simulink model "CrashTest"  (R2024a)
settings: Solver=VariableStepAuto  StartTime=0.0  StopTime=Inf  RelTol=1e-3
model workspace (MAT data in the model file):
  SL_ROS_VariableLengthArrays_MaxSizes.CommonInfo.ArrayTruncateAction = 'EmitWarning'
  SL_ROS_VariableLengthArrays_MaxSizes.MsgTypeMap = containers.Map
  SL_ROS_VariableLengthArrays_MaxSizes.MsgTypeMap.serialization.keys = {'sensor_msgs/PointCloud2', 'sensor_msgs/PointField'}
  SL_ROS_VariableLengthArrays_MaxSizes.MsgTypeMap.serialization.values{1}(1).PropertyName = 'Data'
  SL_ROS_VariableLengthArrays_MaxSizes.MsgTypeMap.serialization.values{1}(1).DataType = 'uint8'
  SL_ROS_VariableLengthArrays_MaxSizes.MsgTypeMap.serialization.values{1}(1).MaxLength = 1000000
  SL_ROS_VariableLengthArrays_MaxSizes.MsgTypeMap.serialization.values{1}(2).PropertyName = 'Fields'
  SL_ROS_VariableLengthArrays_MaxSizes.MsgTypeMap.serialization.values{1}(2).DataType = 'sensor_msgs/PointField'
  SL_ROS_VariableLengthArrays_MaxSizes.MsgTypeMap.serialization.values{1}(2).MaxLength = 16
  SL_ROS_VariableLengthArrays_MaxSizes.MsgTypeMap.serialization.values{2}.PropertyName = 'Name'
  SL_ROS_VariableLengthArrays_MaxSizes.MsgTypeMap.serialization.values{2}.DataType = 'uint8'
  SL_ROS_VariableLengthArrays_MaxSizes.MsgTypeMap.serialization.values{2}.MaxLength = 1000000
  SL_ROS_VariableLengthArrays_MaxSizes.MsgTypeMap.serialization.uniformity = 0
  SL_ROS_VariableLengthArrays_MaxSizes.MsgTypeMap.serialization.keyType = 'char'
  SL_ROS_VariableLengthArrays_MaxSizes.MsgTypeMap.serialization.valueType = 'any'
libraries: robotlib x4, visionsinks x1
settings Model: Creator=lajos  LastModifiedBy=Fahim
settings RTWCC: GPUComputeCapability=3.5

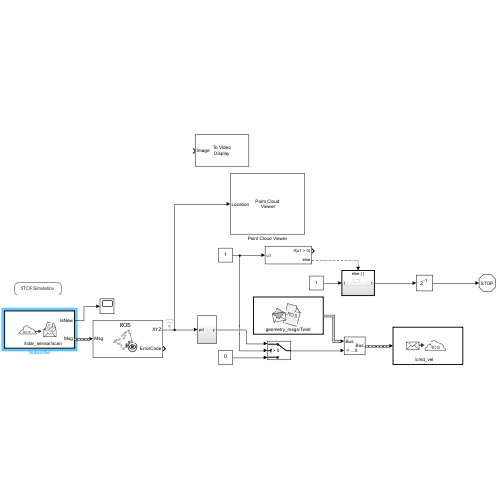
[thumbnail: Simulink's stored preview of the top-level diagram]
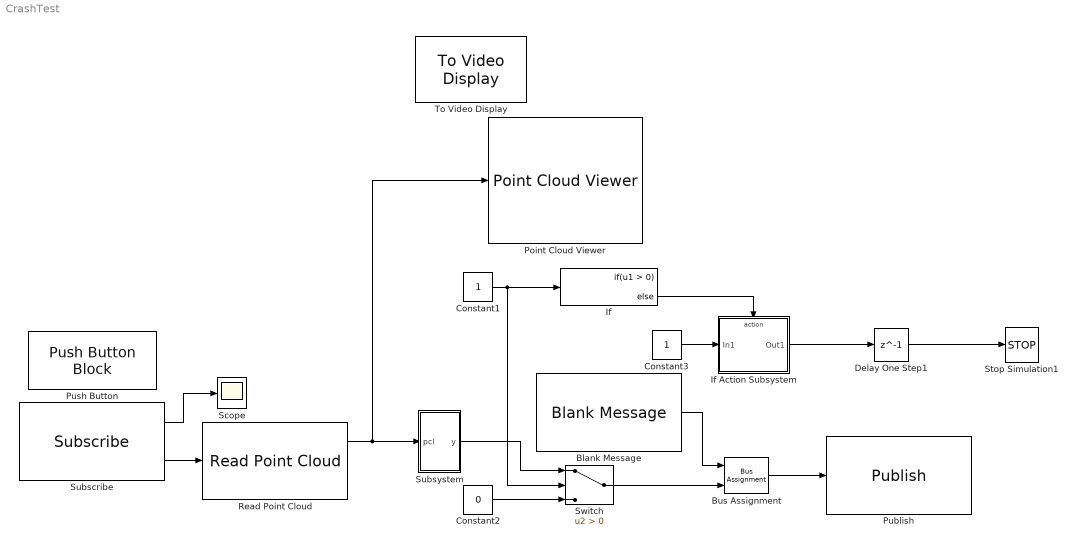
== system CrashTest ==
  Blank Message : robotlib/Blank Message  messageClass=Message  entityType=geometry_msgs/Twist  messageType=geometry_msgs/Twist  SampleTime=inf  legacyBusStruct=off
  Bus Assignment : BusAssignment  AssignedSignals=Linear.X
  Constant1 : Constant
  Constant2 : Constant  Value=0
  Constant3 : Constant
  Delay One Step1 : Delay  DelayLength=1
  If : If  ZeroCross=off
  If Action Subsystem : Subsystem  TreatAsAtomicUnit=on
  Point Cloud Viewer : PointCloudViewer  FigPos=[723 606 410 300]
  Publish : robotlib/Publish  topicSource=Select from ROS network  topic=/cmd_vel  messageType=geometry_msgs/Twist  legacyBusStruct=off  messageQueueLength=1
  Push Button : PushButtonBlock  ButtonText=STOP Simulation  OnValue=0  OffValue=1.000000
  Read Point Cloud : robotlib/Read Point Cloud  MaximumPointCloudSize=[ 100, 3506 ]  PreserveStructure=off  ShowRGBOutput=off  ShowIntensityOutput=off  ShowErrorCodeOutput=on  VariableSizeOutputs=off
  Scope : Scope
  Stop Simulation1 : Stop
  Subscribe : robotlib/Subscribe  topicSource=Specify your own  topic=/lidar_sensor/scan  messageType=sensor_msgs/PointCloud2  SampleTime=-1  legacyBusStruct=off  messageQueueLength=1
  Subsystem : Subsystem
  Switch : Switch  Criteria=u2 > Threshold  SaturateOnIntegerOverflow=off  InputSameDT=off
  To Video Display : visionsinks/To Video Display  windowSizeMode=Normal  openAtMdlStart=on  fullScreen=off  videoWindowX=536805376  videoWindowY=536805376  saveWindowSize=off  videoWindowWidth=2147483647  videoWindowHeight=2147483647  inputColorFormat=RGB  inputType=Obsolete  imagePorts=One multidimensional signal  OutputDevice=On-screen video monitor  dataOrg=Column-major  isWindowOpen=off
  wires:
  Constant1/1 -> Switch/2, If/1
  If/2 -> If Action Subsystem/Action
  Constant2/1 -> Switch/3
  Subsystem/1(y) -> Switch/1
  Delay One Step1/1 -> Stop Simulation1/1
  Subscribe/2 -> Read Point Cloud/1
  Read Point Cloud/1 -> Point Cloud Viewer/1, Subsystem/1(pcl)
  If Action Subsystem/1(Out1) -> Delay One Step1/1
  Constant3/1 -> If Action Subsystem/1(In1)
  Bus Assignment/1 -> Publish/1
  Blank Message/1 -> Bus Assignment/1
  Switch/1 -> Bus Assignment/2
  Subscribe/1 -> Scope/1

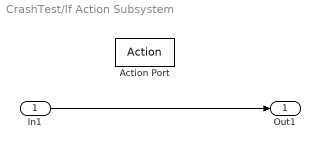
== system CrashTest/If Action Subsystem ==
  In1 : Inport
  Action Port : ActionPort  ActionPortLabel=else
  Out1 : Outport
  wires:
  In1/1 -> Out1/1

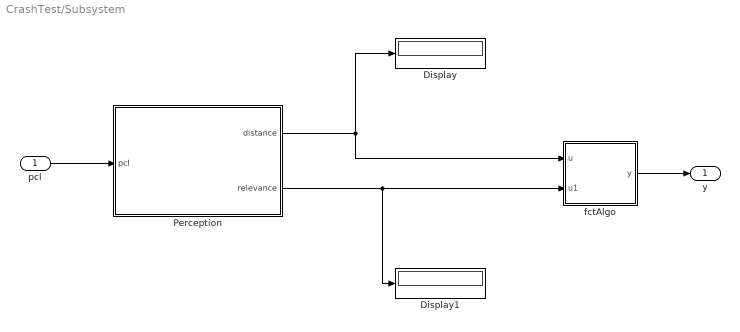
== system CrashTest/Subsystem ==
  pcl : Inport
  Display : Display
  Display1 : Display
  Perception : Subsystem
  fctAlgo : Subsystem
  y : Outport
  wires:
  Perception/2(relevance) -> fctAlgo/2(u1), Display1/1
  fctAlgo/1(y) -> y/1
  Perception/1(distance) -> fctAlgo/1(u), Display/1
  pcl/1 -> Perception/1(pcl)

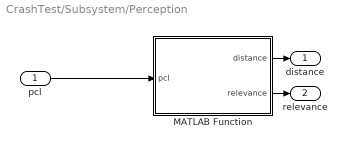
== system CrashTest/Subsystem/Perception ==
  pcl : Inport
  MATLAB Function : MATLAB Function  TreatAsAtomicUnit=on
  distance : Outport
  relevance : Outport  Port=2
  wires:
  pcl/1 -> MATLAB Function/1(pcl)
  MATLAB Function/1(distance) -> distance/1
  MATLAB Function/2(relevance) -> relevance/1

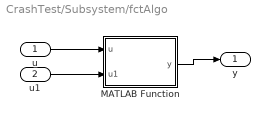
== system CrashTest/Subsystem/fctAlgo ==
  u : Inport
  u1 : Inport  Port=2
  MATLAB Function : MATLAB Function  TreatAsAtomicUnit=on
  y : Outport
  wires:
  u/1 -> MATLAB Function/1(u)
  MATLAB Function/1(y) -> y/1
  u1/1 -> MATLAB Function/2(u1)

== matlab function CrashTest/Subsystem/fctAlgo/MATLAB Function ==
  data: u input; y output; u1 input
function y = fcn(u, u1)

 


y = 1;

== matlab function CrashTest/Subsystem/Perception/MATLAB Function ==
  data: pcl input; distance output; relevance output
function [distance, relevance]  = fcn(pcl)

% Cropping parameters
xmin = -5; 
xmax = 5;
ymin = -1.2;
ymax = 5.2;
zmin = -1.5;
zmax = 10;

xoffset = 0.38; % distance to vehicle front

[row] = find(pcl(:,1) < xmax & pcl(:,1) > xmin & pcl(:,2) > ymin & pcl(:,2) < ymax & pcl(:,3) > zmin & pcl(:,3) < zmax);

tmp = pcl(row,:);

number_of_points = length(tmp);


if number_of_points > 25
    relevance = 1;
    distance = single(mean(tmp(:,1))) - xoffset;
else
    distance = single(5);
    relevance = 0;
end
